simulink model "BD_SER2"  (Simulink 4.1.1)
settings: Solver=ode1  SolverMode=SingleTasking  StartTime=0.0  StopTime=max(cyc_mph(:,1))  FixedStep=1  MaxStep=1  RelTol=1e-3  AbsTol=1e-3
undefined symbols (not defined in the file): air_cp, amb_tmp, cyc_avg_time, cyc_cargo_mass, cyc_elevation_init, cyc_filter_bool, cyc_grade, cyc_mph, enable_stop, ess_cap_scale, ess_coulombic_eff, ess_init_soc, ess_max_ah_cap, ess_max_volts, ess_min_volts, ess_mod_airflow, ess_mod_cp, ess_mod_init_tmp, ess_module_mass, ess_module_num, ess_on, ess_res_scale_coef, ess_res_scale_fun, ess_set_tmp, ess_th_calc, ess_th_res_off, ess_th_res_on, ess_tmp, ess_voc, ex_calc, fc_ct_trq, fc_emis, fc_inertia, fc_map_spd, fc_max_trq, fc_spd_scale, fc_trq_scale, fd_inertia, fd_loss, fd_ratio, gb_dnshift_load, gb_dnshift_spd, gb_gears_num, gb_inertia, gb_num_init, gb_ratio, gb_shift_delay, gb_spd_scale, gb_trq_scale, gb_upshift_load, gb_upshift_spd, gc_inertia, gc_map_spd, gc_map_trq, gc_max_crrnt, gc_max_trq, gc_outpwr_map, gc_overtrq_factor, gc_spd_scale, gc_trq_scale ... (+37)
libraries: lib_wheel2 x12, lib_accessory2 x4, lib_controls2 x3, lib_etc x2, lib_help x2, lib_fuel_converter x2, lib_drive_cycle2 x1, lib_interactive x1, lib_drive_cycle x1, lib_exhaust x1, lib_fuel_converter3 x1
(part 2 of 15)

== system BD_SER2/<cs> control strategy/Motor Controller ==
  Bus Selector : BusSelector  OutputSignals=v_prev  MuxedOutput=off
  Bus Selector1 : BusSelector  OutputSignals=key_on  MuxedOutput=off
  Bus Selector2 : BusSelector  OutputSignals=veh_spd_a_rec  MuxedOutput=off
  Bus Selector3 : BusSelector  OutputSignals=bus_voltage  MuxedOutput=off
  Bus Selector4 : BusSelector  OutputSignals=mpha  MuxedOutput=off
  Bus Selector5 : BusSelector  OutputSignals=cycle_mph_r  MuxedOutput=off
  Bus Selector6 : BusSelector  OutputSignals=current_veh_mass  MuxedOutput=off
  Bus Selector7 : BusSelector  OutputSignals=shifting  MuxedOutput=off
  Constant : Constant  Value=cyc_mph(1,2)*0.447/wh_radius*fd_ratio*gb_ratio(gb_num_init)
  Memory{,1..3} (4 alike) : Memory  X0=ess_module_num*mean(ess_voc(1,:))  InheritSampleTime=off
      settings: RTWStateStorageClass=Auto
  Mux : Mux  Inputs=9
  motor controller : Subsystem
      settings: RTWFcnNameOpts=Auto  RTWFileNameOpts=Auto
  tag scope: mcControl=global
  wires:
  [vehSensors] -> Bus Selector/1
  Bus Selector/1 -> motor controller/1(v_prev in)  "<v_prev>"
  [fcControl] -> Bus Selector1/1
  Bus Selector1/1 -> motor controller/2(key_on in)  "<key_on>"
  [vehSensors] -> Bus Selector2/1
  Bus Selector2/1 -> Memory3/1  "<veh_spd_a_rec>"
  [essSensors] -> Bus Selector3/1
  Bus Selector3/1 -> Memory/1  "<bus_voltage>"
  Memory/1 -> motor controller/4(bus voltage previous)
  [vehSensors] -> Bus Selector4/1
  Bus Selector4/1 -> Memory1/1  "<mpha>"
  [cycReqOut] -> Bus Selector5/1
  Bus Selector5/1 -> Memory2/1  "<cycle_mph_r>"
  [cycSensors] -> Bus Selector6/1
  Bus Selector6/1 -> motor controller/7(current vehicle mass)  "<current_veh_mass>"
  [gbControl] -> Bus Selector7/1
  Bus Selector7/1 -> motor controller/8(shifting)  "<shifting>"
  motor controller/1(v_prev) -> Mux/1  "v_prev"
  motor controller/2(key_on) -> Mux/2  "key_on"
  motor controller/3(veh_spd_a_rec_prev) -> Mux/3  "veh_spd_a_rec_prev"
  motor controller/4(bus_voltage_prev) -> Mux/4  "bus_voltage_prev"
  motor controller/5(mpha_prev) -> Mux/5  "mpha_prev"
  motor controller/6(cyc_mph_r_prev) -> Mux/6  "cyc_mph_r_prev"
  motor controller/7(current_veh_mass) -> Mux/7  "current_veh_mass"
  motor controller/8(shifting out) -> Mux/8  "shifting"
  Mux/1 -> [mcControl]
  motor controller/9(mc_init_spd_est out) -> Mux/9  "mc_init_spd_est"
  Constant/1 -> motor controller/9(mc_init_spd_est)
  Memory1/1 -> motor controller/5(mpha_prev in)
  Memory2/1 -> motor controller/6(cyc_mph_r_prev in)
  Memory3/1 -> motor controller/3(veh_spd_a_rec_prev in)

== system BD_SER2/<cs> control strategy/Power Bus ==
  Constant : Constant  Value=ess_on*1
  power bus controller : Subsystem
      settings: RTWFcnNameOpts=Auto  RTWFileNameOpts=Auto
  tag scope: pbControl=global
  wires:
  power bus controller/1(ess_on) -> [pbControl]
  Constant/1 -> power bus controller/1(enable source two on power bus?)

== system BD_SER2/<cs> control strategy/Wheel Control ==
  Bus Selector : BusSelector  OutputSignals=v_init  MuxedOutput=off
  Bus Selector1 : BusSelector  OutputSignals=current_veh_mass  MuxedOutput=off
  Bus Selector2 : BusSelector  OutputSignals=grade  MuxedOutput=off
  dummy controls : lib_wheel2/vehicle controls/dummy controls
      settings: RTWFcnNameOpts=Auto  RTWFileNameOpts=Auto
  tag scope: vehControl=global
  wires:
  [cycReqOut] -> Bus Selector/1
  Bus Selector/1 -> dummy controls/1  "<v_init>"
  Bus Selector1/1 -> dummy controls/2  "<current_veh_mass>"
  Bus Selector2/1 -> dummy controls/3  "<grade>"
  [cycSensors] -> Bus Selector2/1
  [cycSensors] -> Bus Selector1/1
  dummy controls/1 -> [vehControl]

== system BD_SER2/ACC ELEC <acce>/ACC ELEC model and interface ==
  note: w_APU_speed is used for the speed based electrical loads
      | there shouldn't be any APU speeds (shaft speeds) involved with
      | the electrical accessory case where a power bus is running the loads
      | --see Elec Aux Loads HiV Pwr
  note: MODEL
  note: acc_on Enables/Disables the entire accessory system
  note: INTERFACE
  "requested electrical Power, out to the driveline (W)" : Inport  Port=1  LatchInput=off
  achieved power in from power source (W) : Inport  Port=2  LatchInput=off
  control : Inport  Port=3  LatchInput=off
  Bus Creator : BusCreator  Inputs=2
  Constant : Constant  Value=0
  Demux : Demux  Outputs=4  BusSelectionMode=off
  Goto Tag Visibility1 : GotoTagVisibility  GotoTag=acc_elec_pwr_a
  Goto Tag Visibility11 : GotoTagVisibility  GotoTag=F_req
  Goto Tag Visibility12 : GotoTagVisibility  GotoTag=key_on
  Goto Tag Visibility13 : GotoTagVisibility  GotoTag=engine_on
  Goto Tag Visibility2 : GotoTagVisibility  GotoTag=w_APU_speed
  Goto Tag Visibility3 : GotoTagVisibility  GotoTag=acc_elec_pwr_r
  Goto Tag Visibility9 : GotoTagVisibility  GotoTag=acc_on
  electrical accessory model : Subsystem
      settings: RTWFcnNameOpts=Auto  RTWFileNameOpts=Auto
  signal annotator : Subsystem
      settings: RTWFcnNameOpts=Auto  RTWFileNameOpts=Auto
  requested out : Outport  Port=1
  "requested electrical Power, in from the power source (W)" : Outport  Port=2
  "achieved electrical Power, out to the driveline (W)" : Outport  Port=3
  sensors : Outport  Port=4
  tag scope: F_req=scoped, acc_on=scoped, engine_on=scoped, key_on=scoped, w_APU_speed=scoped
  wires:
  Constant/1 -> [w_APU_speed]
  signal annotator/1(Out1) -> requested out/1
  control/1 -> Demux/1
  Bus Creator/1 -> sensors/1
  Demux/4 -> [engine_on]
  Demux/3 -> [key_on]
  [acc_elec_pwr_a] -> Bus Creator/2  "acc_elec_pwr_a"
  [acc_elec_pwr_r] -> Bus Creator/1  "acc_elec_pwr_r"
  Demux/2 -> [F_req]
  Demux/1 -> [acc_on]
  electrical accessory model/2("achieved electrical Power, out to the driveline (W)") -> "achieved electrical Power, out to the driveline (W)"/1
  achieved power in from power source (W)/1 -> electrical accessory model/2(achieved power in from power source (W))
  electrical accessory model/1("requested electrical Power, in from the power source (W)") -> "requested electrical Power, in from the power source (W)"/1
  "requested electrical Power, out to the driveline (W)"/1 -> signal annotator/1(In1), electrical accessory model/1("requested electrical Power, out to the driveline (W)")

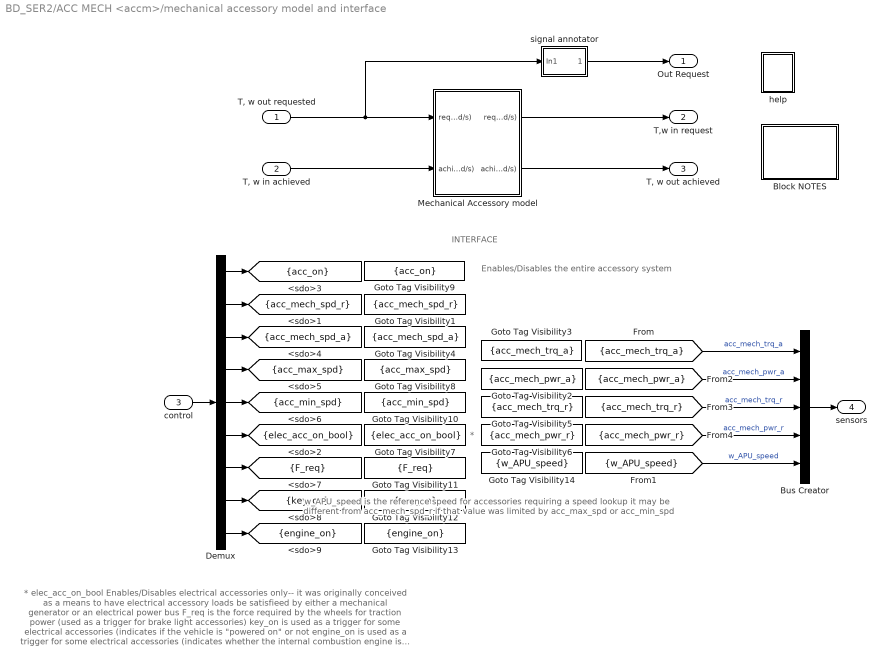
== system BD_SER2/ACC MECH <accm>/mechanical accessory model and interface ==
  note: w_APU_speed is the reference speed for accessories requiring a speed lookup
      | it may be different from acc_mech_spd_r if that value was limited by acc_max_spd
      | or acc_min_spd
  note: * elec_acc_on_bool Enables/Disables electrical accessories only-- it was originally conceived as a means to have electrical accessory loads be
      | satisfieed by either a mechanical generator or an electrical power bus
      |
      | F_req is the force required by the wheels for traction power (used as a trigger for brake light accessories)
      |
      | key_on is used as a trigger for some electrical accessories (indicates if the vehicle is "powered on" or not
      |
      | engine_on is used as a trigger for some electrical accessories (indicates whether the internal combustion engine is running or not) used
      | for starter motor
  note: *
  note: Enables/Disables the entire accessory system
  note: INTERFACE
  "T, w out requested" : Inport  Port=1  LatchInput=off
  "T, w in achieved" : Inport  Port=2  LatchInput=off
  control : Inport  Port=3  LatchInput=off
  Block NOTES : Subsystem
      settings: RTWFcnNameOpts=Auto  RTWFileNameOpts=Auto
      mask Display: disp('Block\nNOTES')
  Bus Creator : BusCreator  Inputs=5
  Demux : Demux  Outputs=9  BusSelectionMode=off
  Goto Tag Visibility1 : GotoTagVisibility  GotoTag=acc_mech_spd_r
  Goto Tag Visibility10 : GotoTagVisibility  GotoTag=acc_min_spd
  Goto Tag Visibility11 : GotoTagVisibility  GotoTag=F_req
  Goto Tag Visibility12 : GotoTagVisibility  GotoTag=key_on
  Goto Tag Visibility13 : GotoTagVisibility  GotoTag=engine_on
  Goto Tag Visibility14 : GotoTagVisibility  GotoTag=w_APU_speed
  Goto Tag Visibility2 : GotoTagVisibility  GotoTag=acc_mech_pwr_a
  Goto Tag Visibility3 : GotoTagVisibility  GotoTag=acc_mech_trq_a
  Goto Tag Visibility4 : GotoTagVisibility  GotoTag=acc_mech_spd_a
  Goto Tag Visibility5 : GotoTagVisibility  GotoTag=acc_mech_trq_r
  Goto Tag Visibility6 : GotoTagVisibility  GotoTag=acc_mech_pwr_r
  Goto Tag Visibility7 : GotoTagVisibility  GotoTag=elec_acc_on_bool
  Goto Tag Visibility8 : GotoTagVisibility  GotoTag=acc_max_spd
  Goto Tag Visibility9 : GotoTagVisibility  GotoTag=acc_on
  Mechanical Accessory model : Subsystem
      settings: RTWFcnNameOpts=Auto  RTWFileNameOpts=Auto
      mask Display: image(imread('bdi_acc_pic.bmp'))
  help : Subsystem
      settings: OpenFcn=web(['file:\\\' which('motor_controller.htm')]);  RTWFcnNameOpts=Auto  RTWFileNameOpts=Auto
      mask Display: image(imread('doc_man.jpg'))
  signal annotator : Subsystem
      settings: RTWFcnNameOpts=Auto  RTWFileNameOpts=Auto
  Out Request : Outport  Port=1
  T,w in request : Outport  Port=2
  "T, w out achieved" : Outport  Port=3
  sensors : Outport  Port=4
  tag scope: F_req=scoped, acc_max_spd=scoped, acc_mech_spd_a=scoped, acc_mech_spd_r=scoped, acc_min_spd=scoped, acc_on=scoped, elec_acc_on_bool=scoped, engine_on=scoped, key_on=scoped
  wires:
  Demux/9 -> [engine_on]
  Demux/8 -> [key_on]
  Demux/7 -> [F_req]
  [w_APU_speed] -> Bus Creator/5  "w_APU_speed"
  Demux/6 -> [elec_acc_on_bool]
  signal annotator/1(Out1) -> Out Request/1
  control/1 -> Demux/1
  Bus Creator/1 -> sensors/1
  Demux/5 -> [acc_min_spd]
  Demux/4 -> [acc_max_spd]
  Demux/3 -> [acc_mech_spd_a]
  [acc_mech_pwr_r] -> Bus Creator/4  "acc_mech_pwr_r"
  [acc_mech_trq_r] -> Bus Creator/3  "acc_mech_trq_r"
  [acc_mech_pwr_a] -> Bus Creator/2  "acc_mech_pwr_a"
  [acc_mech_trq_a] -> Bus Creator/1  "acc_mech_trq_a"
  Demux/2 -> [acc_mech_spd_r]
  Demux/1 -> [acc_on]
  Mechanical Accessory model/2("achieved shaft T and w, out to the driveline (Nm ; rad/s)") -> "T, w out achieved"/1
  "T, w in achieved"/1 -> Mechanical Accessory model/2("achieved shaft and belt T and w, in from the prime mover (Nm ; rad/s)")
  Mechanical Accessory model/1("requested shaft and belt T and w, in from the prime mover (Nm ; rad/s)") -> T,w in request/1
  "T, w out requested"/1 -> signal annotator/1(In1), Mechanical Accessory model/1("requested shaft T and w, out to the driveline  (Nm ; rad/s; rad/s)")

== system BD_SER2/drive cycle <cyc>/drive cycle model and interface ==
  note: DRIVE CYCLE
      | interface
  note: DRIVE CYCLE
      | model
  control : Inport  Port=1  LatchInput=off
  Bus Creator : BusCreator  Inputs=5
  Clock : Clock
      settings: DisplayTime=off  Decimation=10
  Constant : Constant  Value=veh_mass
  Demux : Demux  Outputs=4  BusSelectionMode=off
  Goto Tag Visibility : GotoTagVisibility  GotoTag=mpha
  Goto Tag Visibility1 : GotoTagVisibility  GotoTag=distance
  Goto Tag Visibility10 : GotoTagVisibility  GotoTag=altia_cyc_mph_r
  Goto Tag Visibility2 : GotoTagVisibility  GotoTag=grade_orig
  Goto Tag Visibility3 : GotoTagVisibility  GotoTag=altia_grade
  Goto Tag Visibility4 : GotoTagVisibility  GotoTag=Altia_Run
  Goto Tag Visibility5 : GotoTagVisibility  GotoTag=grade
  Goto Tag Visibility6 : GotoTagVisibility  GotoTag=elevation
  Goto Tag Visibility7 : GotoTagVisibility  GotoTag=veh_cargo_mass
  Goto Tag Visibility8 : GotoTagVisibility  GotoTag=cyc_mph_r_orig
  Goto Tag Visibility9 : GotoTagVisibility  GotoTag=cyc_mph_r
  Sum : Sum  Inputs=++|  SaturateOnIntegerOverflow=on
  drive cycle model : Subsystem
      settings: RTWFcnNameOpts=Auto  RTWFileNameOpts=Auto
  signal annotator : Subsystem
      settings: RTWFcnNameOpts=Auto  RTWFileNameOpts=Auto
  req'd lookups : Outport  Port=1  InitialOutput=0
  req'd vehicle speed (m/s) : Outport  Port=2  InitialOutput=0
  sensors : Outport  Port=3  InitialOutput=0
  tag scope: Altia_Run=scoped, altia_cyc_mph_r=scoped, altia_grade=scoped, mpha=scoped
  wires:
  Sum/1 -> Bus Creator/5  "current_veh_mass"
  Constant/1 -> Sum/2
  [cyc_mph_r] -> signal annotator/3(In3)  "cyc_mph_r"
  [cyc_mph_r_orig] -> signal annotator/2(In2)  "cyc_mph_r_orig"
  [veh_cargo_mass] -> Sum/1  "veh_cargo_mass"
  [elevation] -> Bus Creator/4  "elevation"
  [grade] -> Bus Creator/3  "grade"
  [grade_orig] -> Bus Creator/2  "grade_orig"
  [distance] -> Bus Creator/1  "distance"
  Demux/4 -> [altia_cyc_mph_r]
  Demux/3 -> [Altia_Run]
  Demux/2 -> [altia_grade]
  Demux/1 -> [mpha]
  Bus Creator/1 -> sensors/1
  control/1 -> Demux/1
  signal annotator/1(Out1) -> req'd lookups/1
  Clock/1 -> signal annotator/1(In1)
  drive cycle model/1(req'd vehicle speed (m/s)) -> req'd vehicle speed (m/s)/1

== system BD_SER2/ess config/energy storage <ess> ==
  note: Energy Storage System
  power req'd into bus (W) : Inport  Port=1  LatchInput=off
  Block NOTES : Subsystem
      settings: RTWFcnNameOpts=Auto  RTWFileNameOpts=Auto
      mask Display: disp('Block\nNOTES')
  documentation9 : Subsystem
      settings: OpenFcn=web(['file:\\\' which('energy_storage.htm')]);  RTWFcnNameOpts=Auto  RTWFileNameOpts=Auto
      mask Display: image(imread('doc_man.jpg'))
  energy storage <ess> : Subsystem
      settings: RTWFcnNameOpts=Auto  RTWFileNameOpts=Auto
      mask Display: image(imread('bdi_ess.jpg'))
  power available to bus (W) : Outport  Port=1  InitialOutput=0
  tag scope: essReqOut=global, essSensors=global
  wires:
  energy storage <ess>/3(sensors) -> [essSensors]
  energy storage <ess>/2(power available to bus (W)) -> power available to bus (W)/1
  energy storage <ess>/1(required out) -> [essReqOut]
  [essControl] -> energy storage <ess>/2(control)
  power req'd into bus (W)/1 -> energy storage <ess>/1(power req'd into bus (W))

== system BD_SER2/final drive <fd>/Block NOTES ==
  note: The inertia torque is the input torque required to accelerate the
      | final drive's inertia as measured on the input side.
  note: The loss torque is zero when the gears are not turning,
      | and is applied at the input side of the gear reduction.
  note: This final drive model includes loss data, rotational inertia, and a gear reduction.

== system BD_SER2/final drive <fd>/help ==

== system BD_SER2/final drive <fd>/model&interface ==
  note: Model
  note: Interface
  T & w output request : Inport  Port=1  LatchInput=off
  T & w input achieved : Inport  Port=2  LatchInput=off
  control : Inport  Port=3  LatchInput=off
  Ground : Ground
  Terminator : Terminator
  model : Subsystem
      settings: RTWFcnNameOpts=Auto  RTWFileNameOpts=Auto
  signal annotator : Subsystem
      settings: RTWFcnNameOpts=Auto  RTWFileNameOpts=Auto
  out request : Outport  Port=1  InitialOutput=0
  T & w input request : Outport  Port=2  InitialOutput=0
  T & w output achieved : Outport  Port=3  InitialOutput=0
  sensors : Outport  Port=4  InitialOutput=0
  wires:
  signal annotator/1(Out1) -> out request/1
  control/1 -> Terminator/1
  Ground/1 -> sensors/1
  model/2("torque and speed avail. at output side of final drive (Nm), (rad/s)") -> T & w output achieved/1
  T & w input achieved/1 -> model/2("torque and speed avail. at input side of final drive (Nm), (rad/s)")
  T & w output request/1 -> signal annotator/1(In1), model/1("torque and speed req'd at output side of final drive (Nm), (rad/s)")
  model/1("torque and speed req'd at input side of final drive (Nm), (rad/s)") -> T & w input request/1

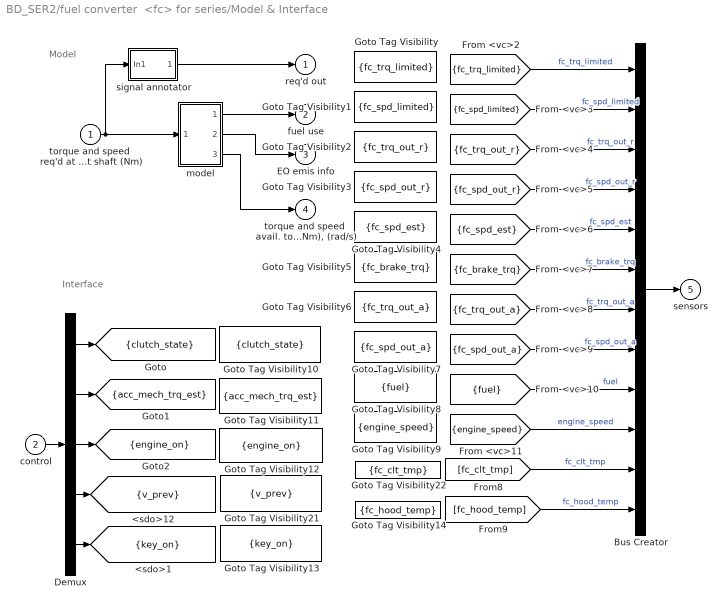
== system BD_SER2/fuel converter  <fc> for series/Model & Interface ==
  note: Interface
  note: Model
  torque and speed  req'd at engine  output shaft (Nm) : Inport  Port=1  LatchInput=off
  control : Inport  Port=2  LatchInput=off
  Bus Creator : BusCreator  Inputs=12
  Demux : Demux  Outputs=5  BusSelectionMode=off
  Goto Tag Visibility : GotoTagVisibility  GotoTag=fc_trq_limited
  Goto Tag Visibility1 : GotoTagVisibility  GotoTag=fc_spd_limited
  Goto Tag Visibility10 : GotoTagVisibility  GotoTag=clutch_state
  Goto Tag Visibility11 : GotoTagVisibility  GotoTag=acc_mech_trq_est
  Goto Tag Visibility12 : GotoTagVisibility  GotoTag=engine_on
  Goto Tag Visibility13 : GotoTagVisibility  GotoTag=key_on
  Goto Tag Visibility14 : GotoTagVisibility  GotoTag=fc_hood_temp
  Goto Tag Visibility2 : GotoTagVisibility  GotoTag=fc_trq_out_r
  Goto Tag Visibility21 : GotoTagVisibility  GotoTag=v_prev
  Goto Tag Visibility22 : GotoTagVisibility  GotoTag=fc_clt_tmp
  Goto Tag Visibility3 : GotoTagVisibility  GotoTag=fc_spd_out_r
  Goto Tag Visibility4 : GotoTagVisibility  GotoTag=fc_spd_est
  Goto Tag Visibility5 : GotoTagVisibility  GotoTag=fc_brake_trq
  Goto Tag Visibility6 : GotoTagVisibility  GotoTag=fc_trq_out_a
  Goto Tag Visibility7 : GotoTagVisibility  GotoTag=fc_spd_out_a
  Goto Tag Visibility8 : GotoTagVisibility  GotoTag=fuel
  Goto Tag Visibility9 : GotoTagVisibility  GotoTag=engine_speed
  model : Subsystem
      settings: RTWFcnNameOpts=Auto  RTWFileNameOpts=Auto
  signal annotator : Subsystem
      settings: RTWFcnNameOpts=Auto  RTWFileNameOpts=Auto
  req'd out : Outport  Port=1  InitialOutput=0
  fuel use : Outport  Port=2  InitialOutput=0
  EO emis info : Outport  Port=3  InitialOutput=0
  "torque and speed  avail. to driveline (Nm), (rad/s)" : Outport  Port=4  InitialOutput=0
  sensors : Outport  Port=5  InitialOutput=0
  tag scope: acc_mech_trq_est=scoped, clutch_state=scoped, engine_on=scoped, key_on=scoped, v_prev=scoped
  wires:
  Demux/5 -> [key_on]
  Demux/4 -> [v_prev]
  [fc_clt_tmp] -> Bus Creator/11  "fc_clt_tmp"
  [fc_hood_temp] -> Bus Creator/12  "fc_hood_temp"
  [engine_speed] -> Bus Creator/10  "engine_speed"
  [fuel] -> Bus Creator/9  "fuel"
  [fc_spd_out_a] -> Bus Creator/8  "fc_spd_out_a"
  [fc_trq_out_a] -> Bus Creator/7  "fc_trq_out_a"
  [fc_brake_trq] -> Bus Creator/6  "fc_brake_trq"
  [fc_spd_est] -> Bus Creator/5  "fc_spd_est"
  [fc_spd_out_r] -> Bus Creator/4  "fc_spd_out_r"
  [fc_trq_out_r] -> Bus Creator/3  "fc_trq_out_r"
  [fc_spd_limited] -> Bus Creator/2  "fc_spd_limited"
  [fc_trq_limited] -> Bus Creator/1  "fc_trq_limited"
  control/1 -> Demux/1
  Demux/3 -> [engine_on]
  Demux/2 -> [acc_mech_trq_est]
  Demux/1 -> [clutch_state]
  Bus Creator/1 -> sensors/1
  signal annotator/1(Out1) -> req'd out/1
  model/3("torque and speed  avail. to driveline (Nm), (rad/s)") -> "torque and speed  avail. to driveline (Nm), (rad/s)"/1
  model/2(EO emis info) -> EO emis info/1
  torque and speed  req'd at engine  output shaft (Nm)/1 -> signal annotator/1(In1), model/1(torque and speed  req'd at engine  output shaft (Nm))
  model/1(fuel use) -> fuel use/1

== system BD_SER2/gearbox <gb> old/Block NOTES ==
  note: This is a good assumption, at least for the VW 4-speed manual transaxle of SAE 820741.
      | In the VW transaxle, efficiency is fairly independent of torque and speed at high torques.
  note: Available output torque is estimated assuming that the gearbox efficiency for theavailable input
      | torque andspeed is the same as the gearbox efficiency for the REQUESTED input torque.
  note: The inertia torque is the input torque required to accelerate the
      | final drive's inertia as measured on the input side.
  note: The loss torque is zero when the gears are not turning,
      | and is applied at the input side of the gear reduction.
  note: This gearbox model includes loss data, rotational inertia, and a gear reduction.

== system BD_SER2/gearbox <gb> old/gearbox model & interface ==
  note: Interface
  note: Model
  trq and spd output request : Inport  Port=1  LatchInput=off
  trq and spd input achieved : Inport  Port=2  LatchInput=off
  controls : Inport  Port=3  LatchInput=off
  Bus Creator : BusCreator  Inputs=5
  Demux2 : Demux  Outputs=3  BusSelectionMode=off
  Goto Tag Visibility : GotoTagVisibility  GotoTag=gear_number
  Goto Tag Visibility1 : GotoTagVisibility  GotoTag=gb_spd_in_a
  Goto Tag Visibility2 : GotoTagVisibility  GotoTag=gear_ratio
  Goto Tag Visibility3 : GotoTagVisibility  GotoTag=shifting
  Goto Tag Visibility4 : GotoTagVisibility  GotoTag=T_gb_out
  Goto Tag Visibility5 : GotoTagVisibility  GotoTag=w_gb_out
  Goto Tag Visibility6 : GotoTagVisibility  GotoTag=eta_gb
  Goto Tag Visibility7 : GotoTagVisibility  GotoTag=gb_trq_out_a
  gearbox model : Subsystem
      settings: RTWFcnNameOpts=Auto  RTWFileNameOpts=Auto
  signal annotator : Subsystem
      settings: RTWFcnNameOpts=Auto  RTWFileNameOpts=Auto
  requested output : Outport  Port=1
  trq and spd input request : Outport  Port=2
  trq and spd output achieved : Outport  Port=3
  sensors : Outport  Port=4
  tag scope: gear_number=scoped, gear_ratio=scoped, shifting=scoped
  wires:
  [gb_trq_out_a] -> Bus Creator/5  "gb_trq_out_a"
  signal annotator/1(Out1) -> requested output/1
  gearbox model/2("torque and speed avail. at output side of gearbox (Nm), (rad/s)") -> trq and spd output achieved/1
  trq and spd input achieved/1 -> gearbox model/2("torque and speed avail. at input side of gearbox (Nm), (rad/s)")
  gearbox model/1("torque and speed req'd at input side of gearbox (Nm), (rad/s)") -> trq and spd input request/1
  trq and spd output request/1 -> signal annotator/1(In1), gearbox model/1("torque and speed req'd at output side of gearbox (Nm), (rad/s)")
  Demux2/3 -> [gear_number]
  Demux2/2 -> [shifting]
  Demux2/1 -> [gear_ratio]
  controls/1 -> Demux2/1
  Bus Creator/1 -> sensors/1
  [eta_gb] -> Bus Creator/4  "eta_gb"
  [w_gb_out] -> Bus Creator/3  "w_gb_out"
  [T_gb_out] -> Bus Creator/2  "T_gb_out"
  [gb_spd_in_a] -> Bus Creator/1  "gb_spd_in_a"

== system BD_SER2/gearbox <gb> old/help ==

== system BD_SER2/generator/ controller <gc>/GC Model ==
  note: Model
  note: Interface
  "torque and speed supplied to rotor (Nm), (rad/s)" : Inport  Port=1  LatchInput=off
  Control : Inport  Port=2  LatchInput=off
  Bus Creator : BusCreator  Inputs=3
  Demux : Demux  Outputs=1  BusSelectionMode=off
  Goto Tag Visibility : GotoTagVisibility  GotoTag=bus_voltage_prev
  Goto Tag Visibility1 : GotoTagVisibility  GotoTag=gc_trq_in_a
  Goto Tag Visibility2 : GotoTagVisibility  GotoTag=gc_spd_in_a
  Goto Tag Visibility3 : GotoTagVisibility  GotoTag=gc_pwr_out_a
  model : Subsystem
      settings: RTWFcnNameOpts=Auto  RTWFileNameOpts=Auto
  signal annotations : Subsystem
      settings: RTWFcnNameOpts=Auto  RTWFileNameOpts=Auto
  requestedOut : Outport  Port=1  InitialOutput=0
  generator output power (W) : Outport  Port=2  InitialOutput=0
  Sensors : Outport  Port=3  InitialOutput=0
  tag scope: bus_voltage_prev=scoped
  wires:
  signal annotations/1(Out1) -> requestedOut/1
  Bus Creator/1 -> Sensors/1
  [gc_pwr_out_a] -> Bus Creator/3
  [gc_spd_in_a] -> Bus Creator/2
  [gc_trq_in_a] -> Bus Creator/1
  Control/1 -> Demux/1
  model/1(generator output power (W)) -> generator output power (W)/1
  "torque and speed supplied to rotor (Nm), (rad/s)"/1 -> signal annotations/1(In1), model/1("torque and speed supplied to rotor (Nm), (rad/s)")
  Demux/1 -> [bus_voltage_prev]

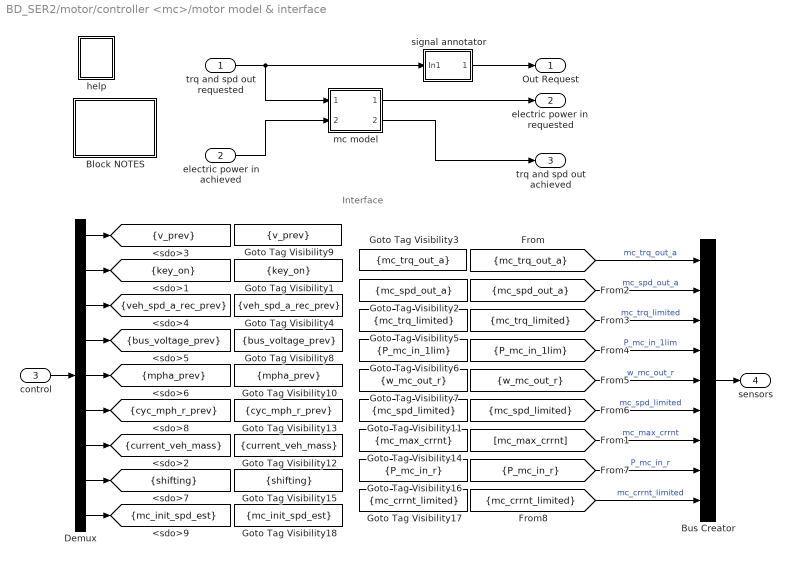
== system BD_SER2/motor/controller <mc>/motor model & interface ==
  note: Interface
  trq and spd out requested : Inport  Port=1  LatchInput=off
  electric power in achieved : Inport  Port=2  LatchInput=off
  control : Inport  Port=3  LatchInput=off
  Block NOTES : Subsystem
      settings: RTWFcnNameOpts=Auto  RTWFileNameOpts=Auto
      mask Display: disp('Block\nNOTES')
  Bus Creator : BusCreator  Inputs=9
  Demux : Demux  Outputs=9  BusSelectionMode=off
  Goto Tag Visibility1 : GotoTagVisibility  GotoTag=key_on
  Goto Tag Visibility10 : GotoTagVisibility  GotoTag=mpha_prev
  Goto Tag Visibility11 : GotoTagVisibility  GotoTag=mc_spd_limited
  Goto Tag Visibility12 : GotoTagVisibility  GotoTag=current_veh_mass
  Goto Tag Visibility13 : GotoTagVisibility  GotoTag=cyc_mph_r_prev
  Goto Tag Visibility14 : GotoTagVisibility  GotoTag=mc_max_crrnt
  Goto Tag Visibility15 : GotoTagVisibility  GotoTag=shifting
  Goto Tag Visibility16 : GotoTagVisibility  GotoTag=P_mc_in_r
  Goto Tag Visibility17 : GotoTagVisibility  GotoTag=mc_crrnt_limited
  Goto Tag Visibility18 : GotoTagVisibility  GotoTag=mc_init_spd_est
  Goto Tag Visibility2 : GotoTagVisibility  GotoTag=mc_spd_out_a
  Goto Tag Visibility3 : GotoTagVisibility  GotoTag=mc_trq_out_a
  Goto Tag Visibility4 : GotoTagVisibility  GotoTag=veh_spd_a_rec_prev
  Goto Tag Visibility5 : GotoTagVisibility  GotoTag=mc_trq_limited
  Goto Tag Visibility6 : GotoTagVisibility  GotoTag=P_mc_in_1lim
  Goto Tag Visibility7 : GotoTagVisibility  GotoTag=w_mc_out_r
  Goto Tag Visibility8 : GotoTagVisibility  GotoTag=bus_voltage_prev
  Goto Tag Visibility9 : GotoTagVisibility  GotoTag=v_prev
  help : Subsystem
      settings: OpenFcn=web(['file:\\\' which('motor_controller.htm')]);  RTWFcnNameOpts=Auto  RTWFileNameOpts=Auto
      mask Display: image(imread('doc_man.jpg'))
  mc model : Subsystem
      settings: RTWFcnNameOpts=Auto  RTWFileNameOpts=Auto
  signal annotator : Subsystem
      settings: RTWFcnNameOpts=Auto  RTWFileNameOpts=Auto
  Out Request : Outport  Port=1
  electric power in  requested : Outport  Port=2
  "trq and spd out achieved " : Outport  Port=3
  sensors : Outport  Port=4
  tag scope: bus_voltage_prev=scoped, current_veh_mass=scoped, cyc_mph_r_prev=scoped, key_on=scoped, mc_init_spd_est=scoped, mpha_prev=scoped, shifting=scoped, v_prev=scoped, veh_spd_a_rec_prev=scoped
  wires:
  [mc_max_crrnt] -> Bus Creator/7  "mc_max_crrnt"
  signal annotator/1(Out1) -> Out Request/1
  control/1 -> Demux/1
  Bus Creator/1 -> sensors/1
  Demux/7 -> [current_veh_mass]
  Demux/6 -> [cyc_mph_r_prev]
  [mc_spd_limited] -> Bus Creator/6  "mc_spd_limited"
  Demux/5 -> [mpha_prev]
  Demux/4 -> [bus_voltage_prev]
  Demux/3 -> [veh_spd_a_rec_prev]
  [w_mc_out_r] -> Bus Creator/5  "w_mc_out_r"
  [P_mc_in_1lim] -> Bus Creator/4  "P_mc_in_1lim"
  [mc_trq_limited] -> Bus Creator/3  "mc_trq_limited"
  [mc_spd_out_a] -> Bus Creator/2  "mc_spd_out_a"
  [mc_trq_out_a] -> Bus Creator/1  "mc_trq_out_a"
  Demux/2 -> [key_on]
  Demux/1 -> [v_prev]
  mc model/2("drive torque and speed avail. at rotor (Nm), (rad/s)") -> "trq and spd out achieved "/1
  mc model/1(req'd motor input power (W)) -> electric power in  requested/1
  electric power in achieved/1 -> mc model/2(available motor input power (W))
  trq and spd out requested/1 -> signal annotator/1(In1), mc model/1("torque and speed  req'd at rotor (Nm), (rad/s)")
  Demux/8 -> [shifting]
  [P_mc_in_r] -> Bus Creator/8  "P_mc_in_r"
  [mc_crrnt_limited] -> Bus Creator/9  "mc_crrnt_limited"
  Demux/9 -> [mc_init_spd_est]

== system BD_SER2/power bus <pb>/Block NOTES ==
  note: This block models the internal combustion engine, and includes inertia effects,
      | performance limits, accessory loads, and temperature transient effects on fuel
      | use, engine-out emissions, and catalyst efficiency.  There are 'leads' to the
      | engine controller here, which controller determines whether the engine is on.

== system BD_SER2/power bus <pb>/help ==

== system BD_SER2/power bus <pb>/power bus ==
  note: Power Bus Model
  note: Interface
  power out req : Inport  Port=1  LatchInput=off
  power available from source one : Inport  Port=2  LatchInput=off
  power available from source two : Inport  Port=3  LatchInput=off
  control : Inport  Port=4  LatchInput=off
  Demux : Demux  Outputs=1  BusSelectionMode=off
  Goto Tag Visibility : GotoTagVisibility  GotoTag=enable_source_two
  Ground : Ground
  model : Subsystem
      settings: RTWFcnNameOpts=Auto  RTWFileNameOpts=Auto
  signal annotator : Subsystem
      settings: RTWFcnNameOpts=Auto  RTWFileNameOpts=Auto
  required out : Outport  Port=1
  power in req from  source one : Outport  Port=2
  power in req from  source two : Outport  Port=3
  power out available : Outport  Port=4
  sensors : Outport  Port=5
  tag scope: enable_source_two=scoped
  wires:
  Ground/1 -> sensors/1
  Demux/1 -> [enable_source_two]
  control/1 -> Demux/1
  signal annotator/1(Out1) -> required out/1
  power available from source two/1 -> model/3(power available from energy storage (W))
  model/3(output power  available at bus) -> power out available/1
  power available from source one/1 -> model/2(power available from generator (W))
  model/2(power req'd from energy storage (W)) -> power in req from  source two/1
  power out req/1 -> signal annotator/1(In1), model/1(req'd power output (W))
  model/1(power req'd from generator (W)) -> power in req from  source one/1

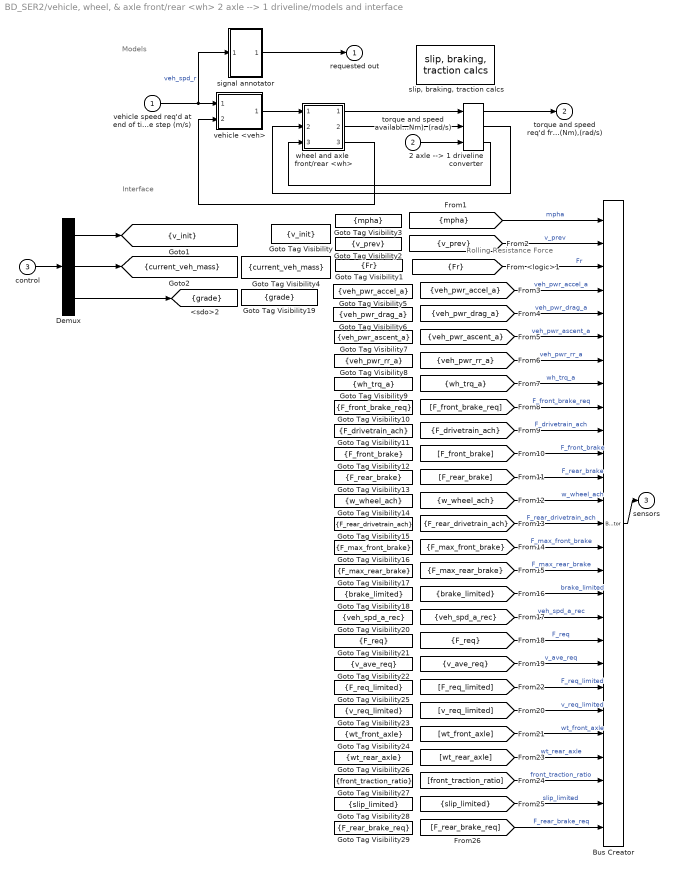
== system BD_SER2/vehicle, wheel, & axle front/rear <wh> 2 axle --> 1 driveline/models and interface ==
  note: Interface
  note: Models
  note: Rolling Resistance Force
  vehicle speed req'd at end of time step (m/s) : Inport  Port=1  LatchInput=off
  "torque and speed available from drivetrain into axles (Nm), (rad/s)" : Inport  Port=2  LatchInput=off
  control : Inport  Port=3  LatchInput=off
  2 axle --> 1 driveline converter : lib_wheel2/Submodels/2 axle --> 1 driveline converter
      settings: RTWFcnNameOpts=Auto  RTWFileNameOpts=Auto
  Bus Creator : BusCreator  Inputs=27
  Demux : Demux  Outputs=3  BusSelectionMode=off
  Goto Tag Visibility : GotoTagVisibility  GotoTag=v_init
  Goto Tag Visibility1 : GotoTagVisibility  GotoTag=Fr
  Goto Tag Visibility10 : GotoTagVisibility  GotoTag=F_front_brake_req
  Goto Tag Visibility11 : GotoTagVisibility  GotoTag=F_drivetrain_ach
  Goto Tag Visibility12 : GotoTagVisibility  GotoTag=F_front_brake
  Goto Tag Visibility13 : GotoTagVisibility  GotoTag=F_rear_brake
  Goto Tag Visibility14 : GotoTagVisibility  GotoTag=w_wheel_ach
  Goto Tag Visibility15 : GotoTagVisibility  GotoTag=F_rear_drivetrain_ach
  Goto Tag Visibility16 : GotoTagVisibility  GotoTag=F_max_front_brake
  Goto Tag Visibility17 : GotoTagVisibility  GotoTag=F_max_rear_brake
  Goto Tag Visibility18 : GotoTagVisibility  GotoTag=brake_limited
  Goto Tag Visibility19 : GotoTagVisibility  GotoTag=grade
  Goto Tag Visibility2 : GotoTagVisibility  GotoTag=v_prev
  Goto Tag Visibility20 : GotoTagVisibility  GotoTag=veh_spd_a_rec
  Goto Tag Visibility21 : GotoTagVisibility  GotoTag=F_req
  Goto Tag Visibility22 : GotoTagVisibility  GotoTag=v_ave_req
  Goto Tag Visibility23 : GotoTagVisibility  GotoTag=v_req_limited
  Goto Tag Visibility24 : GotoTagVisibility  GotoTag=wt_front_axle
  Goto Tag Visibility25 : GotoTagVisibility  GotoTag=F_req_limited
  Goto Tag Visibility26 : GotoTagVisibility  GotoTag=wt_rear_axle
  Goto Tag Visibility27 : GotoTagVisibility  GotoTag=front_traction_ratio
  Goto Tag Visibility28 : GotoTagVisibility  GotoTag=slip_limited
  Goto Tag Visibility29 : GotoTagVisibility  GotoTag=F_rear_brake_req
  Goto Tag Visibility3 : GotoTagVisibility  GotoTag=mpha
  Goto Tag Visibility4 : GotoTagVisibility  GotoTag=current_veh_mass
  Goto Tag Visibility5 : GotoTagVisibility  GotoTag=veh_pwr_accel_a
  Goto Tag Visibility6 : GotoTagVisibility  GotoTag=veh_pwr_drag_a
  Goto Tag Visibility7 : GotoTagVisibility  GotoTag=veh_pwr_ascent_a
  Goto Tag Visibility8 : GotoTagVisibility  GotoTag=veh_pwr_rr_a
  Goto Tag Visibility9 : GotoTagVisibility  GotoTag=wh_trq_a
  signal annotator : Subsystem
      settings: RTWFcnNameOpts=Auto  RTWFileNameOpts=Auto
  "slip, braking, traction calcs" : lib_wheel2/vehicle, wheel, & axle front//rear <wh>/models and interface/slip, braking, traction calcs
      link override config traction control: BlockChoice=traction control 2 axle
      settings: RTWFcnNameOpts=Auto  RTWFileNameOpts=Auto
  vehicle <veh> : Subsystem
      settings: RTWFcnNameOpts=Auto  RTWFileNameOpts=Auto
      mask Display: image(imread('bdi_veh.jpg'))
  wheel and axle  front/rear <wh> : Subsystem
      settings: RTWFcnNameOpts=Auto  RTWFileNameOpts=Auto
      mask Display: image(imread('bdi_wh.jpg'))
  requested out : Outport  Port=1  InitialOutput=0
  torque and speed req'd from drivetrain into axles (Nm),(rad/s) : Outport  Port=2  InitialOutput=0
  sensors : Outport  Port=3  InitialOutput=0
  tag scope: current_veh_mass=scoped, grade=scoped, v_init=scoped
  wires:
  signal annotator/1(Out1) -> requested out/1
  [F_rear_brake_req] -> Bus Creator/27  "F_rear_brake_req"
  [slip_limited] -> Bus Creator/26  "slip_limited"
  2 axle --> 1 driveline converter/1 -> torque and speed req'd from drivetrain into axles (Nm),(rad/s)/1
  2 axle --> 1 driveline converter/3 -> wheel and axle  front/rear <wh>/3("torque and speed available from drivetrain into rear axle (Nm), (rad/s)")
  2 axle --> 1 driveline converter/2 -> wheel and axle  front/rear <wh>/2("torque and speed available from drivetrain into front axle (Nm), (rad/s)")
  "torque and speed available from drivetrain into axles (Nm), (rad/s)"/1 -> 2 axle --> 1 driveline converter/3
  [front_traction_ratio] -> Bus Creator/25  "front_traction_ratio"
  [wt_rear_axle] -> Bus Creator/24  "wt_rear_axle"
  [wt_front_axle] -> Bus Creator/23  "wt_front_axle"
  [v_req_limited] -> Bus Creator/22  "v_req_limited"
  [F_req_limited] -> Bus Creator/21  "F_req_limited"
  [v_ave_req] -> Bus Creator/20  "v_ave_req"
  [F_req] -> Bus Creator/19  "F_req"
  [veh_spd_a_rec] -> Bus Creator/18  "veh_spd_a_rec"
  [brake_limited] -> Bus Creator/17  "brake_limited"
  [F_max_rear_brake] -> Bus Creator/16  "F_max_rear_brake"
  [F_max_front_brake] -> Bus Creator/15  "F_max_front_brake"
  [F_rear_drivetrain_ach] -> Bus Creator/14  "F_rear_drivetrain_ach"
  [w_wheel_ach] -> Bus Creator/13  "w_wheel_ach"
  [F_rear_brake] -> Bus Creator/12  "F_rear_brake"
  [F_front_brake] -> Bus Creator/11  "F_front_brake"
  [F_drivetrain_ach] -> Bus Creator/10  "F_drivetrain_ach"
  [F_front_brake_req] -> Bus Creator/9  "F_front_brake_req"
  [wh_trq_a] -> Bus Creator/8  "wh_trq_a"
  [veh_pwr_rr_a] -> Bus Creator/7  "veh_pwr_rr_a"
  [veh_pwr_ascent_a] -> Bus Creator/6  "veh_pwr_ascent_a"
  [veh_pwr_drag_a] -> Bus Creator/5  "veh_pwr_drag_a"
  [veh_pwr_accel_a] -> Bus Creator/4  "veh_pwr_accel_a"
  [v_prev] -> Bus Creator/2  "v_prev"
  [mpha] -> Bus Creator/1  "mpha"
  Bus Creator/1 -> sensors/1
  [Fr] -> Bus Creator/3  "Fr"
  Demux/3 -> [grade]
  Demux/2 -> [current_veh_mass]
  Demux/1 -> [v_init]
  control/1 -> Demux/1
  wheel and axle  front/rear <wh>/2(torque and speed req'd from drivetrain into rear axle (Nm),(rad/s)) -> 2 axle --> 1 driveline converter/2
  wheel and axle  front/rear <wh>/1(torque and speed req'd from drivetrain into front axle (Nm),(rad/s)) -> 2 axle --> 1 driveline converter/1
  wheel and axle  front/rear <wh>/3(tractive force and linear speed  achievable) -> vehicle <veh>/2(tractive force and linear speed achievable (N))
  vehicle <veh>/1("tractive force and speed required of tire and wheel (N), (m/s)") -> wheel and axle  front/rear <wh>/1("tractive force and speed req'd of tire/road interface (N), (m/s)")
  vehicle speed req'd at end of time step (m/s)/1 -> vehicle <veh>/1(vehicle speed req'd at end of time step (m/s)), signal annotator/1(veh_spd_r)  "veh_spd_r"

== system BD_SER2/<cs> control strategy/Electrical Accessories/electrical accessory controller ==
  electrical accessories on? : Inport  Port=1  LatchInput=off
  F_req in : Inport  Port=2  LatchInput=off
  key_on in : Inport  Port=3  LatchInput=off
  engine_on in : Inport  Port=4  LatchInput=off
  acc_on : Outport  Port=1  InitialOutput=0
  F_req : Outport  Port=2  InitialOutput=0
  key_on : Outport  Port=3  InitialOutput=0
  engine_on : Outport  Port=4  InitialOutput=0
  wires:
  electrical accessories on?/1 -> acc_on/1  "acc_on"
  engine_on in/1 -> engine_on/1  "engine_on"
  F_req in/1 -> F_req/1  "F_req"
  key_on in/1 -> key_on/1  "key_on"

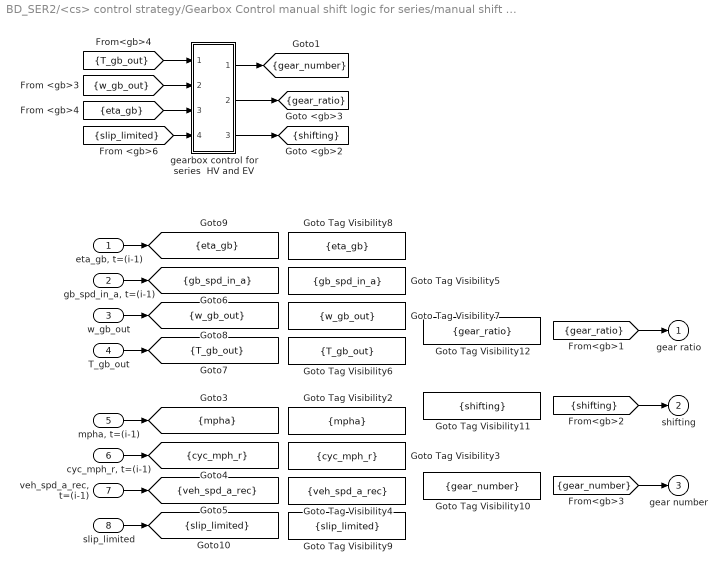
== system BD_SER2/<cs> control strategy/Gearbox Control manual shift logic for series/manual shift logic for series ==
  "eta_gb, t=(i-1)" : Inport  Port=1  LatchInput=off
  "gb_spd_in_a, t=(i-1)" : Inport  Port=2  LatchInput=off
  w_gb_out : Inport  Port=3  LatchInput=off
  T_gb_out : Inport  Port=4  LatchInput=off
  "mpha, t=(i-1)" : Inport  Port=5  LatchInput=off
  "cyc_mph_r, t=(i-1)" : Inport  Port=6  LatchInput=off
  "veh_spd_a_rec, t=(i-1)" : Inport  Port=7  LatchInput=off
  slip_limited : Inport  Port=8  LatchInput=off
  Goto Tag Visibility10 : GotoTagVisibility  GotoTag=gear_number
  Goto Tag Visibility11 : GotoTagVisibility  GotoTag=shifting
  Goto Tag Visibility12 : GotoTagVisibility  GotoTag=gear_ratio
  Goto Tag Visibility2 : GotoTagVisibility  GotoTag=mpha
  Goto Tag Visibility3 : GotoTagVisibility  GotoTag=cyc_mph_r
  Goto Tag Visibility4 : GotoTagVisibility  GotoTag=veh_spd_a_rec
  Goto Tag Visibility5 : GotoTagVisibility  GotoTag=gb_spd_in_a
  Goto Tag Visibility6 : GotoTagVisibility  GotoTag=T_gb_out
  Goto Tag Visibility7 : GotoTagVisibility  GotoTag=w_gb_out
  Goto Tag Visibility8 : GotoTagVisibility  GotoTag=eta_gb
  Goto Tag Visibility9 : GotoTagVisibility  GotoTag=slip_limited
  gearbox control for series  HV and EV : Subsystem
      settings: RTWFcnNameOpts=Auto  RTWFileNameOpts=Auto
  gear ratio : Outport  Port=1  InitialOutput=0
  shifting : Outport  Port=2  InitialOutput=0
  gear number : Outport  Port=3  InitialOutput=0
  tag scope: T_gb_out=scoped, cyc_mph_r=scoped, eta_gb=scoped, gb_spd_in_a=scoped, gear_number=scoped, gear_ratio=scoped, mpha=scoped, shifting=scoped, slip_limited=scoped, veh_spd_a_rec=scoped, w_gb_out=scoped
  wires:
  T_gb_out/1 -> [T_gb_out]
  w_gb_out/1 -> [w_gb_out]
  "gb_spd_in_a, t=(i-1)"/1 -> [gb_spd_in_a]
  [gear_number] -> gear number/1
  [shifting] -> shifting/1
  [gear_ratio] -> gear ratio/1
  slip_limited/1 -> [slip_limited]
  "eta_gb, t=(i-1)"/1 -> [eta_gb]
  "veh_spd_a_rec, t=(i-1)"/1 -> [veh_spd_a_rec]
  "cyc_mph_r, t=(i-1)"/1 -> [cyc_mph_r]
  "mpha, t=(i-1)"/1 -> [mpha]
  [slip_limited] -> gearbox control for series  HV and EV/4(tires are at traction limit)
  [T_gb_out] -> gearbox control for series  HV and EV/1(gb_trq_out_r)
  [w_gb_out] -> gearbox control for series  HV and EV/2(gb_spd_out_r)
  [eta_gb] -> gearbox control for series  HV and EV/3(prev. Pout/Pin)
  gearbox control for series  HV and EV/1("gear number, out") -> [gear_number]
  gearbox control for series  HV and EV/2("gear ratio, out") -> [gear_ratio]
  gearbox control for series  HV and EV/3("shifting, out") -> [shifting]

== system BD_SER2/<cs> control strategy/Generator/generator controller ==
  bus voltage previous in : Inport  Port=1  LatchInput=off
  bus voltage previous out : Outport  Port=1  InitialOutput=0
  wires:
  bus voltage previous in/1 -> bus voltage previous out/1  "bus_voltage"

== system BD_SER2/<cs> control strategy/Hybrid Control Strategy/hybrid controls ==
  ess_max_pwr : Inport  Port=1  LatchInput=off
  SOC : Inport  Port=2  LatchInput=off
  ess_max_chg_pwr : Inport  Port=3  LatchInput=off
  key_on : Inport  Port=4  LatchInput=off
  ess_max_pwr out : Outport  Port=1  InitialOutput=0
  SOC in : Outport  Port=2  InitialOutput=0
  ess_max_chg_pwr out : Outport  Port=3  InitialOutput=0
  key_on out : Outport  Port=4  InitialOutput=0
  wires:
  ess_max_pwr/1 -> ess_max_pwr out/1  "ess_max_pwr"
  SOC/1 -> SOC in/1
  ess_max_chg_pwr/1 -> ess_max_chg_pwr out/1
  key_on/1 -> key_on out/1

== system BD_SER2/<cs> control strategy/IC Engine Control Series Hybrid/Fuel Converter Control ==
  note: Controls for Series Fuel Converter
  note: This is just to give a matching FROM block for the sensors
  engine_on in : Inport  Port=1  LatchInput=off
  acc_mech_trq_est : Inport  Port=2  LatchInput=off
  fcSensors : Inport  Port=3  LatchInput=off
  v_prev : Inport  Port=4  LatchInput=off
  Terminator : Terminator
  key_on : Subsystem  mask(Repeating table){@1=vc_key_on(:,1), @2=vc_key_on(:,2)}
      mask prompts: @1 "Time values:"; @2 "Output values:"
      mask help:
      | Repeating table.
      | Enter values of time and output for first cycle.
      mask init:
      | period = max(@1); t = @1; y = @2;
      settings: RTWFcnNameOpts=Auto  RTWFileNameOpts=Auto
      mask Help: Repeats cycle given in table. Time values should be monotonically increasing.
  series 'clutch' control : Subsystem
      settings: RTWFcnNameOpts=Auto  RTWFileNameOpts=Auto
  clutch state out : Outport  Port=1
  acc_mech_trq_est out : Outport  Port=2
  engine_on out : Outport  Port=3
  v_prev out : Outport  Port=4
  key_on out : Outport  Port=5
  wires:
  fcSensors/1 -> Terminator/1
  series 'clutch' control/1(clutch state) -> clutch state out/1  "clutch_state"
  acc_mech_trq_est/1 -> acc_mech_trq_est out/1  "acc_mech_trq_est"
  v_prev/1 -> v_prev out/1  "v_prev"
  key_on/1(out_1) -> key_on out/1  "key_on"
  engine_on in/1 -> series 'clutch' control/1(engine on), engine_on out/1  "engine_on"

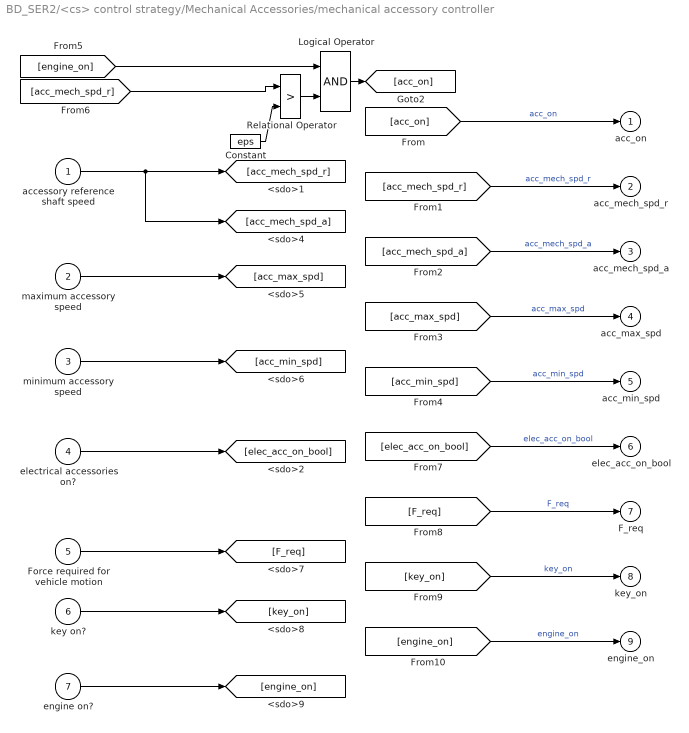
== system BD_SER2/<cs> control strategy/Mechanical Accessories/mechanical accessory controller ==
  accessory reference shaft speed : Inport  Port=1  LatchInput=off
  maximum accessory speed : Inport  Port=2  LatchInput=off
  minimum accessory speed : Inport  Port=3  LatchInput=off
  electrical accessories on? : Inport  Port=4  LatchInput=off
  Force required for vehicle motion : Inport  Port=5  LatchInput=off
  key on? : Inport  Port=6  LatchInput=off
  engine on? : Inport  Port=7  LatchInput=off
  Constant : Constant  Value=eps
  Logical Operator : Logic  Operator=AND  Inputs=2
  Relational Operator : RelationalOperator  Operator=>
  acc_on : Outport  Port=1  InitialOutput=0
  acc_mech_spd_r : Outport  Port=2  InitialOutput=0
  acc_mech_spd_a : Outport  Port=3  InitialOutput=0
  acc_max_spd : Outport  Port=4  InitialOutput=0
  acc_min_spd : Outport  Port=5  InitialOutput=0
  elec_acc_on_bool : Outport  Port=6  InitialOutput=0
  F_req : Outport  Port=7  InitialOutput=0
  key_on : Outport  Port=8  InitialOutput=0
  engine_on : Outport  Port=9  InitialOutput=0
  wires:
  accessory reference shaft speed/1 -> [acc_mech_spd_r], [acc_mech_spd_a]
  maximum accessory speed/1 -> [acc_max_spd]
  minimum accessory speed/1 -> [acc_min_spd]
  electrical accessories on?/1 -> [elec_acc_on_bool]
  Force required for vehicle motion/1 -> [F_req]
  key on?/1 -> [key_on]
  engine on?/1 -> [engine_on]
  [acc_mech_spd_r] -> Relational Operator/1
  Constant/1 -> Relational Operator/2
  [engine_on] -> Logical Operator/1
  Relational Operator/1 -> Logical Operator/2
  Logical Operator/1 -> [acc_on]
  [acc_on] -> acc_on/1  "acc_on"
  [engine_on] -> engine_on/1  "engine_on"
  [key_on] -> key_on/1  "key_on"
  [F_req] -> F_req/1  "F_req"
  [elec_acc_on_bool] -> elec_acc_on_bool/1  "elec_acc_on_bool"
  [acc_min_spd] -> acc_min_spd/1  "acc_min_spd"
  [acc_max_spd] -> acc_max_spd/1  "acc_max_spd"
  [acc_mech_spd_a] -> acc_mech_spd_a/1  "acc_mech_spd_a"
  [acc_mech_spd_r] -> acc_mech_spd_r/1  "acc_mech_spd_r"

== system BD_SER2/<cs> control strategy/Motor Controller/motor controller ==
  v_prev in : Inport  Port=1  LatchInput=off
  key_on in : Inport  Port=2  LatchInput=off
  veh_spd_a_rec_prev in : Inport  Port=3  LatchInput=off
  bus voltage previous : Inport  Port=4  LatchInput=off
  mpha_prev in : Inport  Port=5  LatchInput=off
  cyc_mph_r_prev in : Inport  Port=6  LatchInput=off
  current vehicle mass : Inport  Port=7  LatchInput=off
  shifting : Inport  Port=8  LatchInput=off
  mc_init_spd_est : Inport  Port=9  LatchInput=off
  v_prev : Outport  Port=1
  key_on : Outport  Port=2
  veh_spd_a_rec_prev : Outport  Port=3
  bus_voltage_prev : Outport  Port=4
  mpha_prev : Outport  Port=5
  cyc_mph_r_prev : Outport  Port=6
  current_veh_mass : Outport  Port=7
  shifting out : Outport  Port=8
  mc_init_spd_est out : Outport  Port=9
  wires:
  bus voltage previous/1 -> bus_voltage_prev/1
  v_prev in/1 -> v_prev/1
  key_on in/1 -> key_on/1
  veh_spd_a_rec_prev in/1 -> veh_spd_a_rec_prev/1
  mpha_prev in/1 -> mpha_prev/1
  cyc_mph_r_prev in/1 -> cyc_mph_r_prev/1
  current vehicle mass/1 -> current_veh_mass/1
  shifting/1 -> shifting out/1
  mc_init_spd_est/1 -> mc_init_spd_est out/1

== system BD_SER2/<cs> control strategy/Power Bus/power bus controller ==
  enable source two on power bus? : Inport  Port=1  LatchInput=off
  ess_on : Outport  Port=1
  wires:
  enable source two on power bus?/1 -> ess_on/1
